simulink model "PMSM_sim"  (R2023a)
settings: Solver=ode45  StartTime=0  StopTime=10.0  MaxStep=Max_step_size  RelTol=Relative_tolerance
undefined symbols (not defined in the file or in its folder): f_filter, filter_on, Hm, Ib, id_ref, k_friction, KI_d, KI_q, KI_w, Kp_d, Kp_q, Kp_w, Lb, ld, Ld, lq, Lq, phi, phi_pu, phib, pp, rs, sig_i, sig_w, stair_factor, stair_ramp_selector, t_step, Tb, Tl_cost, Vb, wb, wm_n, wm_slope
libraries: slpidlib x3, simulink x1, spsStairGeneratorLib x1
settings Model: Creator=Juri  LastModifiedBy=mattd
settings DataIOCC: SignalLogging=off

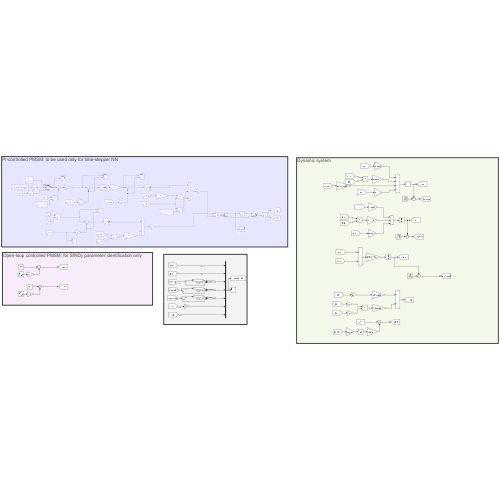
[thumbnail: Simulink's stored preview of the top-level diagram]
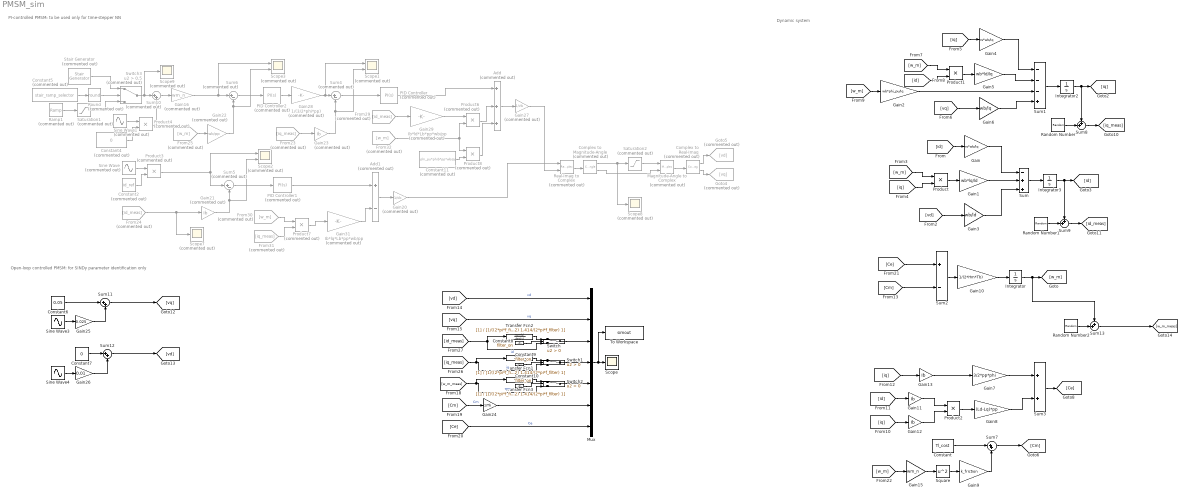
== system PMSM_sim ==
  note: Dynamic system
  note: Open-loop controlled PMSM: for SINDy parameter identification only
  note: PI-controlled PMSM: to be used only for time-stepper NN
  Add : Sum  Commented=on  Inputs=+++
  Add1 : Sum  Commented=on  Inputs=+-
  Complex to Magnitude-Angle : ComplexToMagnitudeAngle  Commented=on
  Complex to Real-Imag : ComplexToRealImag  Commented=on
  Constant : Constant  Value=Tl_cost
  Constant10 : Constant  Value=filter_on
  Constant11 : Constant  Commented=on  Value=phi_pu*phib*pp*wb/pp
  Constant2 : Constant  Commented=on  Value=id_ref
  Constant4 : Constant  Commented=on  Value=0
  Constant5 : Constant  Commented=on  Value=stair_ramp_selector
  Constant6 : Constant  Value=0.05
  Constant7 : Constant  Value=0
  Constant8 : Constant  Value=filter_on
  Constant9 : Constant  Value=filter_on
  From23 : From  Commented=on  GotoTag=iq_meas
  From24 : From  Commented=on  GotoTag=id_meas
  From25 : From  Commented=on  GotoTag=w_m
  From29 : From  Commented=on  GotoTag=id_meas
  From30 : From  Commented=on  GotoTag=w_m
  From31 : From  Commented=on  GotoTag=iq_meas
  From32 : From  Commented=on  GotoTag=w_m
  Gain : Gain  Gain=rs*wb/lq
  Gain1 : Gain  Gain=wb*lq/ld
  Gain10 : Gain  Gain=1/(2*Hm*Tb)
  Gain11 : Gain  Gain=Ib
  Gain12 : Gain  Gain=Ib
  Gain13 : Gain  Gain=Ib
  Gain15 : Gain  Gain=wm_n
  Gain16 : Gain  Commented=on  Gain=wm_n
  Gain2 : Gain  Gain=wb*phi_pu/lq
  Gain20 : Gain  Commented=on  Gain=1/Vb
  Gain21 : Gain  Commented=on  Gain=Ib
  Gain22 : Gain  Commented=on  Gain=wb/pp
  Gain23 : Gain  Commented=on  Gain=Ib
  Gain24 : Gain  Gain=1/Tb
  Gain25 : Gain  Gain=0.025
  Gain26 : Gain  Gain=0.01
  Gain27 : Gain  Commented=on  Gain=1/Vb
  Gain28 : Gain  Commented=on  Gain=1/(3/2*phi*pp)
  Gain29 : Gain  Commented=on  Gain=Ib*ld*Lb*pp*wb/pp
  Gain3 : Gain  Gain=wb/ld
  Gain31 : Gain  Commented=on  Gain=Ib*lq*Lb*pp*wb/pp
  Gain4 : Gain  Gain=rs*wb/lq
  Gain5 : Gain  Gain=wb*ld/lq
  Gain6 : Gain  Gain=wb/lq
  Gain7 : Gain  Gain=3/2*pp*phi
  Gain8 : Gain  Gain=(Ld-Lq)*pp
  Gain9 : Gain  Gain=k_friction
  Goto4 : Goto  Commented=on  GotoTag=vq
  Goto5 : Goto  Commented=on  GotoTag=vd
  Integrator : Integrator
  Integrator2 : Integrator
  Integrator3 : Integrator
  Magnitude-Angle to Complex : MagnitudeAngleToComplex  Commented=on
  Mux : Mux  Inputs=7
  PID Controller : slpidlib/PID Controller  Commented=on  Controller=PI  Form=Parallel  TimeDomain=Continuous-time  UseExternalTs=off  SampleTime=-1  IntegratorMethod=Forward Euler  FilterMethod=Forward Euler  ControllerParametersSource=internal  P=Kp_q  I=KI_q  UseKiTs=off  D=0  N=100  UseFilter=on  TunerSelectOption=Transfer Function Based (PID Tuner App)  InitialConditionSource=internal  InitialConditionForIntegrator=0  InitialConditionForFilter=0  DifferentiatorICPrevScaledInput=0  ExternalReset=none  TrackingMode=off  Kt=1  LimitOutput=on  SatLimitsSource=internal  UpperSaturationLimit=Vb  LowerSaturationLimit=-Vb  LinearizeAsGain=on  AntiWindupMode=clamping  Kb=1  LimitIntegrator=off  UpperIntegratorSaturationLimit=inf  LowerIntegratorSaturationLimit=-inf  POutMin=[]  POutMax=[]  IOutMin=[]  IOutMax=[]  DOutMin=[]  DOutMax=[]  NOutMin=[]  NOutMax=[]  SumOutMin=[]  SumOutMax=[]  SaturationOutMin=[]  SaturationOutMax=[]  PParamMin=[]  PParamMax=[]  IParamMin=[]  IParamMax=[]  DParamMin=[]  DParamMax=[]  NParamMin=[]  NParamMax=[]  KbParamMin=[]  KbParamMax=[]  KtParamMin=[]  KtParamMax=[]  KbOutMin=[]  KbOutMax=[]  KtOutMin=[]  KtOutMax=[]  IntegratorOutMin=[]  IntegratorOutMax=[]  FilterOutMin=[]  FilterOutMax=[]  SumI1OutMin=[]  SumI1OutMax=[]  SumI2OutMin=[]  SumI2OutMax=[]  SumI3OutMin=[]  SumI3OutMax=[]  SumI4OutMin=[]  SumI4OutMax=[]  SumDOutMin=[]  SumDOutMax=[]  DifferentiatorOutMin=[]  DifferentiatorOutMax=[]  FilterDiffOutCoefMin=[]  FilterDiffOutCoefMax=[]  ReciprocalOutMin=[]  ReciprocalOutMax=[]  SumDenOutMin=[]  SumDenOutMax=[]  SumNumOutMin=[]  SumNumOutMax=[]  DivideOutMin=[]  DivideOutMax=[]  UdiffTsProdOutMin=[]  UdiffTsProdOutMax=[]  NTsProdOutMin=[]  NTsProdOutMax=[]  UintegralTsProdOutMin=[]  UintegralTsProdOutMax=[]  UngainTsProdOutMin=[]  UngainTsProdOutMax=[]  ClampingZeroOutDataTypeStr=Inherit: Inherit via back propagation  ClampingZeroOutMin=[]  ClampingZeroOutMax=[]  FilterDenConstantOutDataTypeStr=Inherit: Inherit via back propagation  FilterDenConstantOutMin=[]  FilterDenConstantOutMax=[]  PCopyOutDataTypeStr=Inherit: Inherit via back propagation  PCopyOutMin=[]  PCopyOutMax=[]  NCopyOutDataTypeStr=Inherit: Inherit via back propagation  NCopyOutMin=[]  NCopyOutMax=[]  IntegratorContinuousStateAttributes=''  IntegratorStateMustResolveToSignalObject=off  IntegratorRTWStateStorageClass=Auto  FilterContinuousStateAttributes=''  FilterStateMustResolveToSignalObject=off  FilterRTWStateStorageClass=Auto  ParallelPVariant=InternalParameters  IdealPVariant=Disabled  IVariant=InternalParameters  DVariant=Disabled  IntegratorVariant=Continuous  SatVariant=Enabled  AWVariant=ContClampingParallel  PCopyVariant=Disabled  TRVariant=Disabled  FdbkBlocksVariant=Forward  IdealPFdbkVariant=Disabled  SatFdbkVariant=Disabled  DerivativeFilterVariant=Disabled  NVariant=Disabled  NCopyVariant=Disabled_SignalSpec  FilterICVariant=Disabled  IntegratorICVariant=InternalICs  ExternalResetVariant=Disabled  TRSumVariant=Passthrough  SumFdbkVariant=Disabled  SumVariant=Sum_PI  TsampFilterVariant=InternalTs  TsampNgainVariant=Passthrough  TsampIntegralVariant=Disabled_SignalSpec  ExternalSaturationOutDataTypeStr=Inherit: Same as second input
  PID Controller1 : slpidlib/PID Controller  Commented=on  Controller=PI  Form=Parallel  TimeDomain=Continuous-time  UseExternalTs=off  SampleTime=-1  IntegratorMethod=Forward Euler  FilterMethod=Forward Euler  ControllerParametersSource=internal  P=Kp_d  I=KI_d  UseKiTs=off  D=0  N=100  UseFilter=on  TunerSelectOption=Transfer Function Based (PID Tuner App)  InitialConditionSource=internal  InitialConditionForIntegrator=0  InitialConditionForFilter=0  DifferentiatorICPrevScaledInput=0  ExternalReset=none  TrackingMode=off  Kt=1  LimitOutput=on  SatLimitsSource=internal  UpperSaturationLimit=Vb  LowerSaturationLimit=-Vb  LinearizeAsGain=on  AntiWindupMode=clamping  Kb=1  LimitIntegrator=off  UpperIntegratorSaturationLimit=inf  LowerIntegratorSaturationLimit=-inf  POutMin=[]  POutMax=[]  IOutMin=[]  IOutMax=[]  DOutMin=[]  DOutMax=[]  NOutMin=[]  NOutMax=[]  SumOutMin=[]  SumOutMax=[]  SaturationOutMin=[]  SaturationOutMax=[]  PParamMin=[]  PParamMax=[]  IParamMin=[]  IParamMax=[]  DParamMin=[]  DParamMax=[]  NParamMin=[]  NParamMax=[]  KbParamMin=[]  KbParamMax=[]  KtParamMin=[]  KtParamMax=[]  KbOutMin=[]  KbOutMax=[]  KtOutMin=[]  KtOutMax=[]  IntegratorOutMin=[]  IntegratorOutMax=[]  FilterOutMin=[]  FilterOutMax=[]  SumI1OutMin=[]  SumI1OutMax=[]  SumI2OutMin=[]  SumI2OutMax=[]  SumI3OutMin=[]  SumI3OutMax=[]  SumI4OutMin=[]  SumI4OutMax=[]  SumDOutMin=[]  SumDOutMax=[]  DifferentiatorOutMin=[]  DifferentiatorOutMax=[]  FilterDiffOutCoefMin=[]  FilterDiffOutCoefMax=[]  ReciprocalOutMin=[]  ReciprocalOutMax=[]  SumDenOutMin=[]  SumDenOutMax=[]  SumNumOutMin=[]  SumNumOutMax=[]  DivideOutMin=[]  DivideOutMax=[]  UdiffTsProdOutMin=[]  UdiffTsProdOutMax=[]  NTsProdOutMin=[]  NTsProdOutMax=[]  UintegralTsProdOutMin=[]  UintegralTsProdOutMax=[]  UngainTsProdOutMin=[]  UngainTsProdOutMax=[]  ClampingZeroOutDataTypeStr=Inherit: Inherit via back propagation  ClampingZeroOutMin=[]  ClampingZeroOutMax=[]  FilterDenConstantOutDataTypeStr=Inherit: Inherit via back propagation  FilterDenConstantOutMin=[]  FilterDenConstantOutMax=[]  PCopyOutDataTypeStr=Inherit: Inherit via back propagation  PCopyOutMin=[]  PCopyOutMax=[]  NCopyOutDataTypeStr=Inherit: Inherit via back propagation  NCopyOutMin=[]  NCopyOutMax=[]  IntegratorContinuousStateAttributes=''  IntegratorStateMustResolveToSignalObject=off  IntegratorRTWStateStorageClass=Auto  FilterContinuousStateAttributes=''  FilterStateMustResolveToSignalObject=off  FilterRTWStateStorageClass=Auto  ParallelPVariant=InternalParameters  IdealPVariant=Disabled  IVariant=InternalParameters  DVariant=Disabled  IntegratorVariant=Continuous  SatVariant=Enabled  AWVariant=ContClampingParallel  PCopyVariant=Disabled  TRVariant=Disabled  FdbkBlocksVariant=Forward  IdealPFdbkVariant=Disabled  SatFdbkVariant=Disabled  DerivativeFilterVariant=Disabled  NVariant=Disabled  NCopyVariant=Disabled_SignalSpec  FilterICVariant=Disabled  IntegratorICVariant=InternalICs  ExternalResetVariant=Disabled  TRSumVariant=Passthrough  SumFdbkVariant=Disabled  SumVariant=Sum_PI  TsampFilterVariant=InternalTs  TsampNgainVariant=Passthrough  TsampIntegralVariant=Disabled_SignalSpec  ExternalSaturationOutDataTypeStr=Inherit: Same as second input
  PID Controller2 : slpidlib/PID Controller  Commented=on  Controller=PI  Form=Parallel  TimeDomain=Continuous-time  UseExternalTs=off  SampleTime=-1  IntegratorMethod=Forward Euler  FilterMethod=Forward Euler  ControllerParametersSource=internal  P=Kp_w  I=KI_w  UseKiTs=off  D=0  N=100  UseFilter=on  TunerSelectOption=Transfer Function Based (PID Tuner App)  InitialConditionSource=internal  InitialConditionForIntegrator=0  InitialConditionForFilter=0  DifferentiatorICPrevScaledInput=0  ExternalReset=none  TrackingMode=off  Kt=1  LimitOutput=on  SatLimitsSource=internal  UpperSaturationLimit=Tb  LowerSaturationLimit=-Tb  LinearizeAsGain=on  AntiWindupMode=clamping  Kb=1  LimitIntegrator=off  UpperIntegratorSaturationLimit=inf  LowerIntegratorSaturationLimit=-inf  POutMin=[]  POutMax=[]  IOutMin=[]  IOutMax=[]  DOutMin=[]  DOutMax=[]  NOutMin=[]  NOutMax=[]  SumOutMin=[]  SumOutMax=[]  SaturationOutMin=[]  SaturationOutMax=[]  PParamMin=[]  PParamMax=[]  IParamMin=[]  IParamMax=[]  DParamMin=[]  DParamMax=[]  NParamMin=[]  NParamMax=[]  KbParamMin=[]  KbParamMax=[]  KtParamMin=[]  KtParamMax=[]  KbOutMin=[]  KbOutMax=[]  KtOutMin=[]  KtOutMax=[]  IntegratorOutMin=[]  IntegratorOutMax=[]  FilterOutMin=[]  FilterOutMax=[]  SumI1OutMin=[]  SumI1OutMax=[]  SumI2OutMin=[]  SumI2OutMax=[]  SumI3OutMin=[]  SumI3OutMax=[]  SumI4OutMin=[]  SumI4OutMax=[]  SumDOutMin=[]  SumDOutMax=[]  DifferentiatorOutMin=[]  DifferentiatorOutMax=[]  FilterDiffOutCoefMin=[]  FilterDiffOutCoefMax=[]  ReciprocalOutMin=[]  ReciprocalOutMax=[]  SumDenOutMin=[]  SumDenOutMax=[]  SumNumOutMin=[]  SumNumOutMax=[]  DivideOutMin=[]  DivideOutMax=[]  UdiffTsProdOutMin=[]  UdiffTsProdOutMax=[]  NTsProdOutMin=[]  NTsProdOutMax=[]  UintegralTsProdOutMin=[]  UintegralTsProdOutMax=[]  UngainTsProdOutMin=[]  UngainTsProdOutMax=[]  ClampingZeroOutDataTypeStr=Inherit: Inherit via back propagation  ClampingZeroOutMin=[]  ClampingZeroOutMax=[]  FilterDenConstantOutDataTypeStr=Inherit: Inherit via back propagation  FilterDenConstantOutMin=[]  FilterDenConstantOutMax=[]  PCopyOutDataTypeStr=Inherit: Inherit via back propagation  PCopyOutMin=[]  PCopyOutMax=[]  NCopyOutDataTypeStr=Inherit: Inherit via back propagation  NCopyOutMin=[]  NCopyOutMax=[]  IntegratorContinuousStateAttributes=''  IntegratorStateMustResolveToSignalObject=off  IntegratorRTWStateStorageClass=Auto  FilterContinuousStateAttributes=''  FilterStateMustResolveToSignalObject=off  FilterRTWStateStorageClass=Auto  ParallelPVariant=InternalParameters  IdealPVariant=Disabled  IVariant=InternalParameters  DVariant=Disabled  IntegratorVariant=Continuous  SatVariant=Enabled  AWVariant=ContClampingParallel  PCopyVariant=Disabled  TRVariant=Disabled  FdbkBlocksVariant=Forward  IdealPFdbkVariant=Disabled  SatFdbkVariant=Disabled  DerivativeFilterVariant=Disabled  NVariant=Disabled  NCopyVariant=Disabled_SignalSpec  FilterICVariant=Disabled  IntegratorICVariant=InternalICs  ExternalResetVariant=Disabled  TRSumVariant=Passthrough  SumFdbkVariant=Disabled  SumVariant=Sum_PI  TsampFilterVariant=InternalTs  TsampNgainVariant=Passthrough  TsampIntegralVariant=Disabled_SignalSpec  ExternalSaturationOutDataTypeStr=Inherit: Same as second input
  Product : Product
  Product1 : Product
  Product2 : Product
  Product{3..4,6..8} (5 alike) : Product  Commented=on
  Ramp1 : simulink/Sources/Ramp  Commented=on  slope=wm_slope  start=0  InitialOutput=0
  Random Number : RandomNumber  Variance=sig_i  SampleTime=t_step/10
  Random Number1 : RandomNumber  Variance=sig_i  SampleTime=t_step/10
  Random Number2 : RandomNumber  Variance=sig_w  SampleTime=t_step/10
  Real-Imag to Complex : RealImagToComplex  Commented=on
  Round : Rounding  Commented=on  Operator=round
  Saturation1 : Saturate  Commented=on  UpperLimit=0.4
  Saturation2 : Saturate  Commented=on  UpperLimit=1  LowerLimit=-1
  Scope : Scope
  Scope1 : Scope  Commented=on  NumInputPorts=2
  Scope2 : Scope  Commented=on  NumInputPorts=2
  Scope3 : Scope  Commented=on  NumInputPorts=2
  Scope7 : Scope  Commented=on
  Scope8 : Scope  Commented=on
  Scope9 : Scope  Commented=on
  Sine Wave : Sin  Commented=on  Frequency=2*pi  SampleTime=0
  Sine Wave1 : Sin  Commented=on  Frequency=2*pi  SampleTime=0
  Sine Wave3 : Sin  Frequency=2*pi*0.1  SampleTime=0
  Sine Wave4 : Sin  Frequency=2*pi*5  SampleTime=0
  Square : Math  Operator=square
  Stair Generator : spsStairGeneratorLib/Stair Generator  Commented=on  t=[0,1e-3, 2, 4, 6, 8]  e=[0 , 0.1, 0.3, 0.6, 0.8, 0.45].*stair_factor  Ts=0
  Sum : Sum  Inputs=-++
  Sum1 : Sum  Inputs=---+
  Sum10 : Sum  Commented=on  Inputs=|++
  Sum11 : Sum  Inputs=|++
  Sum12 : Sum  Inputs=|++
  Sum13 : Sum  Inputs=++|
  Sum2 : Sum  Inputs=+-
  Sum3 : Sum
  Sum4 : Sum  Commented=on  Inputs=|+-
  Sum5 : Sum  Commented=on  Inputs=|+-
  Sum6 : Sum  Commented=on  Inputs=|+-
  Sum7 : Sum  Inputs=|++
  Sum8 : Sum  Inputs=++|
  Sum9 : Sum  Inputs=++|
  Switch : Switch  Criteria=u2 > Threshold  SaturateOnIntegerOverflow=off  InputSameDT=off
  Switch1 : Switch  Criteria=u2 > Threshold  SaturateOnIntegerOverflow=off  InputSameDT=off
  Switch2 : Switch  Criteria=u2 > Threshold  SaturateOnIntegerOverflow=off  InputSameDT=off
  Switch3 : Switch  Commented=on  Criteria=u2 > Threshold  Threshold=0.5  SaturateOnIntegerOverflow=off  InputSameDT=off
  To Workspace : ToWorkspace  VariableName=simout  SampleTime=t_step
  Transfer Fcn1 : TransferFcn  Denominator=[1/((2*pi*f_filter)^2) 1.414/(2*pi*f_filter) 1]
  Transfer Fcn2 : TransferFcn  Denominator=[1/((2*pi*f_filter)^2) 1.414/(2*pi*f_filter) 1]
  Transfer Fcn3 : TransferFcn  Denominator=[1/((2*pi*f_filter)^2) 1.414/(2*pi*f_filter) 1]
  wires:
  Integrator/1 -> Sum13/1, [w_m]
  Integrator2/1 -> Sum8/1, [iq]
  Sum/1 -> Integrator3/1
  Gain/1 -> Sum/1
  Gain1/1 -> Sum/2
  Gain3/1 -> Sum/3
  [vd] -> Gain3/1
  [id] -> Gain/1
  Product/1 -> Gain1/1
  [w_m] -> Product/1
  [iq] -> Product/2
  [id] -> Product1/2
  [w_m] -> Product1/1
  Product1/1 -> Gain5/1
  [iq] -> Gain4/1
  [vq] -> Gain6/1
  Gain5/1 -> Sum1/2
  Gain4/1 -> Sum1/1
  Gain6/1 -> Sum1/4
  Gain2/1 -> Sum1/3
  [w_m] -> Gain2/1
  Sum1/1 -> Integrator2/1
  Sum2/1 -> Gain10/1
  Product2/1 -> Gain8/1
  [iq] -> Gain12/1
  [id] -> Gain11/1
  [iq] -> Gain13/1
  [Cm] -> Sum2/2
  Mux/1 -> To Workspace/1, Scope/1
  [vd] -> Mux/1  "vd"
  [vq] -> Mux/2  "vq"
  [Cm] -> Gain24/1  "Cm"
  [Ce] -> Mux/7  "Ce"
  [Ce] -> Sum2/1
  Gain7/1 -> Sum3/1
  Gain8/1 -> Sum3/2
  Sum3/1 -> [Ce]
  PID Controller/1 -> Add/1
  Sum4/1 -> PID Controller/1
  From23/1 -> Gain23/1
  From24/1 -> Scope7/1, Gain21/1
  Sum5/1 -> PID Controller1/1
  Product3/1 -> Sum5/1, Scope2/1
  PID Controller2/1 -> Gain28/1
  From25/1 -> Gain22/1
  Sum6/1 -> PID Controller2/1
  [w_m] -> Gain15/1
  Square/1 -> Gain9/1
  Gain9/1 -> Sum7/2
  Gain10/1 -> Integrator/1
  Constant/1 -> Sum7/1
  Sum7/1 -> [Cm]
  Gain11/1 -> Product2/1
  Gain12/1 -> Product2/2
  Gain13/1 -> Gain7/1
  Gain21/1 -> Sum5/2, Scope2/2
  Gain22/1 -> Scope3/2, Sum6/2
  Gain23/1 -> Scope1/2, Sum4/2
  Gain15/1 -> Square/1
  Gain16/1 -> Scope3/1, Sum6/1
  Sine Wave/1 -> Product3/1
  Constant2/1 -> Product3/2
  Random Number/1 -> Sum8/2
  Random Number1/1 -> Sum9/2
  Integrator3/1 -> Sum9/1, [id]
  Gain24/1 -> Mux/6
  Constant4/1 -> Product4/2
  Sine Wave1/1 -> Product4/1
  Product4/1 -> Sum10/2
  Sum10/1 -> Gain16/1
  Constant6/1 -> Sum11/1
  Sine Wave3/1 -> Gain25/1
  Gain25/1 -> Sum11/2
  Constant7/1 -> Sum12/1
  Gain26/1 -> Sum12/2
  Sine Wave4/1 -> Gain26/1
  Sum12/1 -> [vd]
  Sum11/1 -> [vq]
  Random Number2/1 -> Sum13/2
  Sum9/1 -> [id_meas]
  Sum13/1 -> [w_m_meas]
  Constant8/1 -> Switch/2
  Transfer Fcn2/1 -> Switch/1
  [id_meas] -> Transfer Fcn2/1, Switch/3  "id"
  Switch/1 -> Mux/3
  [iq_meas] -> Transfer Fcn1/1, Switch1/3  "iq"
  Transfer Fcn1/1 -> Switch1/1
  Constant9/1 -> Switch1/2
  Constant10/1 -> Switch2/2
  Transfer Fcn3/1 -> Switch2/1
  [w_m_meas] -> Switch2/3, Transfer Fcn3/1  "wm"
  Switch2/1 -> Mux/5
  Switch1/1 -> Mux/4
  Gain28/1 -> Scope1/1, Sum4/1
  Constant11/1 -> Product8/2
  From29/1 -> Gain29/1
  Product6/1 -> Add/2
  Product8/1 -> Add/3
  From32/1 -> Product8/1, Product6/2
  Gain29/1 -> Product6/1
  Product7/1 -> Gain31/1
  From31/1 -> Product7/2
  From30/1 -> Product7/1
  Gain31/1 -> Add1/2
  PID Controller1/1 -> Add1/1
  Add/1 -> Gain27/1
  Add1/1 -> Gain20/1
  Complex to Magnitude-Angle/1 -> Scope8/1, Saturation2/1
  Complex to Real-Imag/2 -> Goto4/1
  Real-Imag to Complex/1 -> Complex to Magnitude-Angle/1
  Magnitude-Angle to Complex/1 -> Complex to Real-Imag/1
  Complex to Real-Imag/1 -> Goto5/1
  Saturation2/1 -> Magnitude-Angle to Complex/1
  Complex to Magnitude-Angle/2 -> Magnitude-Angle to Complex/2
  Gain20/1 -> Real-Imag to Complex/1
  Gain27/1 -> Real-Imag to Complex/2
  Ramp1/1 -> Saturation1/1
  Switch3/1 -> Scope9/1, Sum10/1
  Saturation1/1 -> Switch3/3
  Round/1 -> Switch3/2
  Constant5/1 -> Round/1
  Stair Generator/1 -> Switch3/1
  Sum8/1 -> [iq_meas]
